simulink model "gm_uz_sixphase_VSD_transformation"  (R2021b)
settings: Solver=FixedStepAuto  StartTime=0.0  StopTime=inf  RelTol=1e-3
undefined symbols (not defined in the file or in its folder): a, b, c
libraries: hdlsllib x42, simulink x26, hdlmdlgenlib x20, dspsigops x6
(part 2 of 4)

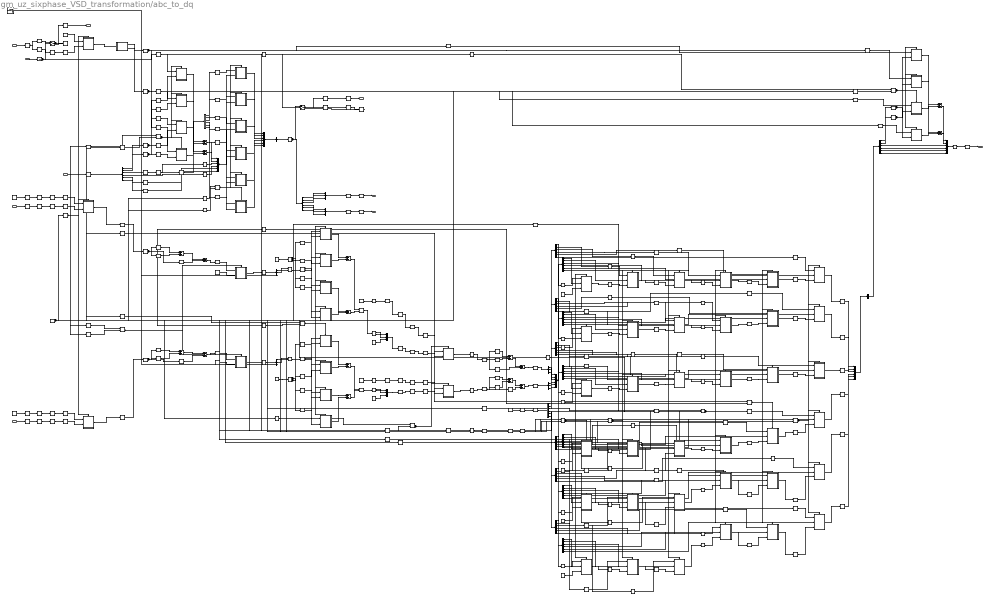
== system gm_uz_sixphase_VSD_transformation/abc_to_dq ==
  note: sin/cos calculation
  note: VSD and Park transformation
  note: VSD and Park inverse transformation
  note: Trigger Output
  x_in_dq : Inport  OutDataTypeStr=fixdt(1, 27, 18)  PortDimensions=[6]  SampleTime=1e-08
  theta_el : Inport  Port=2  OutDataTypeStr=fixdt(1, 18, 14)  PortDimensions=1  SampleTime=1e-08
  trigger_new_values : Inport  Port=3  OutDataTypeStr=boolean  PortDimensions=1  SampleTime=1e-08
  x_abc1_ll_pl : Inport  Port=4  OutDataTypeStr=fixdt(1, 27, 16)  PortDimensions=[3]  SampleTime=1e-08
  x_abc2_ll_pl : Inport  Port=5  OutDataTypeStr=fixdt(1, 27, 16)  PortDimensions=[3]  SampleTime=1e-08
  Add : Sum  AccumDataTypeStr=fixdt(1, 28, 16)  OutDataTypeStr=fixdt(1, 27, 16)  SampleTime=1e-10
  Add1 : Sum  AccumDataTypeStr=fixdt(1, 28, 18)  OutDataTypeStr=fixdt(1, 27, 18)  SampleTime=1e-10
  Add11 : Sum  Inputs=+-  AccumDataTypeStr=fixdt(1, 28, 16)  OutDataTypeStr=fixdt(1, 27, 16)  SampleTime=1e-10
  Add2 : Sum  Inputs=+-  AccumDataTypeStr=fixdt(1, 28, 18)  OutDataTypeStr=fixdt(1, 27, 18)  SampleTime=1e-10
  Complex to Real-Imag : ComplexToRealImag  SampleTime=1e-10
  Complex to Real-Imag1 : ComplexToRealImag  SampleTime=1e-10
  Constant : Constant  Value=0  OutDataTypeStr=fixdt(1, 27, 16)  SampleTime=1e-10
  Constant1 : Constant  Value=[1;-0.5;-0.5;0.86602783203125;-0.86602783203125;0;0;0.86602783203125;-0.86602783203125;0.5;0.5;-1;1;-0.5;-0.5;-0.86602783203125;0.86602783203125;0;0;-0.86602783203125;0.86602783203125;0.5;0.5;-1;1;1;1;0;0;0;0;0;0;1;1;1]  OutDataTypeStr=fixdt(1, 18, 16)  SampleTime=1e-10
  Constant11 : Constant  Value=[0.33333587646484375;0;0.33333587646484375;0;0.33333587646484375;0;-0.16666412353515625;0.28867340087890625;-0.16666412353515625;-0.28867340087890625;0.33333587646484375;0;-0.16666412353515625;-0.28867340087890625;-0.16666412353515625;0.28867340087890625;0.33333587646484375;0;0.28867340087890625;0.16666412353515625;-0.28867340087890625;0.16666412353515625;0;0.33333587646484375;-0.28867340087890625;0.16666412353515625;0.28867340087890625;0.16666412353515625;0;0.33333587646484375;0;-0.33333587646484375;0;-0.33333587646484375;0;0.33333587646484375]  OutDataTypeStr=fixdt(1, 18, 17)  SampleTime=1e-10
  Constant12 : Constant  Value="fi(0,1,18,16,\"hex\",\"08000 + 3b619 i\")"  OutDataTypeStr=fixdt(1, 18, 16)  SampleTime=1e-10
  Constant13 : Constant  Value="fi(0,1,18,16,\"hex\",\"08000 + 3b619 i\")"  OutDataTypeStr=fixdt(1, 18, 16)  SampleTime=1e-10
  Constant2 : Constant  Value=0  OutDataTypeStr=fixdt(1, 27, 16)  SampleTime=1e-10
  Delay9 : RateTransition  OutPortSampleTimeOpt=Multiple of input port sample time  OutPortSampleTimeMultiple=100
  Demux1_mux_1 : Mux  Inputs=3
  Demux1_mux_2 : Mux  Inputs=3
  Demux1_out1 : Delay  DelayLength=double(1)  InitialCondition=0  SampleTime=1e-10
  Demux1_out2 : Delay  DelayLength=double(1)  InitialCondition=0  SampleTime=1e-10
  Divide : Subsystem
      settings: MinAlgLoopOccurrences=on
  Divide1 : Subsystem
      settings: MinAlgLoopOccurrences=on
  Divide11 : Subsystem
      settings: MinAlgLoopOccurrences=on
  Divide2 : Subsystem
      settings: MinAlgLoopOccurrences=on
  Divide21 : Subsystem
      settings: MinAlgLoopOccurrences=on
  Divide3 : Subsystem
      settings: MinAlgLoopOccurrences=on
  Divide31 : Subsystem
      settings: MinAlgLoopOccurrences=on
  Divide4 : Subsystem
      settings: MinAlgLoopOccurrences=on
  From{,1..3,11..12,17..18,21..22} (10 alike) : hdlmdlgenlib/Buffer
      settings: SourceProductBaseCode=SL
  Gain : Subsystem
      settings: MinAlgLoopOccurrences=on
  Gain2 : Subsystem
      settings: MinAlgLoopOccurrences=on
  Gain21 : Subsystem
      settings: MinAlgLoopOccurrences=on
  Gain2_const : Constant  Value=0.6666717529296875  OutDataTypeStr=fixdt(1, 18, 16)  SampleTime=1e-10
  Gain2_const1 : Constant  Value=0.6666717529296875  OutDataTypeStr=fixdt(1, 18, 16)  SampleTime=1e-10
  Gain2_out_dtc : DataTypeConversion  OutDataTypeStr=fixdt(1, 27, 16)  SampleTime=1e-10  SaturateOnIntegerOverflow=on
  Gain2_out_dtc1 : DataTypeConversion  OutDataTypeStr=fixdt(1, 27, 16)  SampleTime=1e-10  SaturateOnIntegerOverflow=on
  Gain4_const : Constant  Value=[1;0;0.5;-0.5;0.86602783203125;0.5;-0.5;-0.86602783203125;0.5]  OutDataTypeStr=fixdt(1, 18, 16)  SampleTime=1e-10
  Gain4_const1 : Constant  Value=[1;-0.5;-0.5;0;0.86602783203125;-0.86602783203125;1;1;1]  OutDataTypeStr=fixdt(1, 18, 16)  SampleTime=1e-10
  Gain4_const2 : Constant  Value=[1;0;0.5;-0.5;0.86602783203125;0.5;-0.5;-0.86602783203125;0.5]  OutDataTypeStr=fixdt(1, 18, 16)  SampleTime=1e-10
  Gain4_const3 : Constant  Value=[1;-0.5;-0.5;0;0.86602783203125;-0.86602783203125;1;1;1]  OutDataTypeStr=fixdt(1, 18, 16)  SampleTime=1e-10
  Gain_const : Constant  Value=0.1591548919677734375  OutDataTypeStr=fixdt(1, 18, 19)  SampleTime=1e-10
  Goto : hdlmdlgenlib/Buffer
      settings: SourceProductBaseCode=SL
  Goto1 : hdlmdlgenlib/Buffer
      settings: SourceProductBaseCode=SL
  Goto2 : hdlmdlgenlib/Buffer
      settings: SourceProductBaseCode=SL
  MMul_add_01 : Sum  OutDataTypeStr=fixdt(1, 27, 16)  SaturateOnIntegerOverflow=on  SampleTime=1e-10
  MMul_add_011 : Sum  OutDataTypeStr=fixdt(1, 27, 16)  SaturateOnIntegerOverflow=on  SampleTime=1e-10
  MMul_add_012 : Sum  OutDataTypeStr=fixdt(1, 27, 16)  SaturateOnIntegerOverflow=on  SampleTime=1e-10
  MMul_add_013 : Sum  OutDataTypeStr=fixdt(1, 27, 16)  SaturateOnIntegerOverflow=on  SampleTime=1e-10
  MMul_add_{12,121..123} (4 alike) : Sum  OutDataTypeStr=fixdt(1, 27, 16)  SaturateOnIntegerOverflow=on  SampleTime=1e-10
  MMul_dot_product : Subsystem
      settings: MinAlgLoopOccurrences=on
  MMul_dot_product1 : Subsystem
      settings: MinAlgLoopOccurrences=on
  MMul_dot_product2 : Subsystem
      settings: MinAlgLoopOccurrences=on
  MMul_dot_product3 : Subsystem
      settings: MinAlgLoopOccurrences=on
  MMul_dot_product_out_dtc{,1..3} (4 alike) : DataTypeConversion  OutDataTypeStr=fixdt(1, 27, 16)  SampleTime=1e-10  SaturateOnIntegerOverflow=on
  MatrixMultiply_out1_0_wire : hdlmdlgenlib/Buffer
      settings: SourceProductBaseCode=SL
  MatrixMultiply_out1_1_wire : hdlmdlgenlib/Buffer
      settings: SourceProductBaseCode=SL
  Product : Subsystem
      settings: MinAlgLoopOccurrences=on
  Product1 : Subsystem
      settings: MinAlgLoopOccurrences=on
  Product2 : Subsystem
      settings: MinAlgLoopOccurrences=on
  Product3 : Subsystem
      settings: MinAlgLoopOccurrences=on
  Product4 : Subsystem
      settings: MinAlgLoopOccurrences=on
  Product5 : Subsystem
      settings: MinAlgLoopOccurrences=on
  Product6 : Subsystem
      settings: MinAlgLoopOccurrences=on
  Product7 : Subsystem
      settings: MinAlgLoopOccurrences=on
  Product_AC_minus_BD : Sum  Inputs=+-  OutDataTypeStr=fixdt(1, 27, 16)  SampleTime=1e-10
  Product_AC_minus_BD1 : Sum  Inputs=+-  OutDataTypeStr=fixdt(1, 27, 16)  SampleTime=1e-10
  Product_AD_plus_BC : Sum  OutDataTypeStr=fixdt(1, 27, 16)  SampleTime=1e-10
  Product_AD_plus_BC1 : Sum  OutDataTypeStr=fixdt(1, 27, 16)  SampleTime=1e-10
  Product_C2ReIm_{1..2,11,21} (4 alike) : ComplexToRealImag  SampleTime=1e-10
  Product_ReIm2Complex : RealImagToComplex  SampleTime=1e-10
  Product_ReIm2Complex1 : RealImagToComplex  SampleTime=1e-10
  Real-Imag to Complex : RealImagToComplex  ConstantPart="fi(0,1,27,16,\"hex\",\"0000000\")"  SampleTime=1e-10
  Real-Imag to Complex1 : RealImagToComplex  ConstantPart="fi(0,1,27,16,\"hex\",\"0000000\")"  SampleTime=1e-10
  Reshape{,1..3} (4 alike) : Reshape  OutputDimensionality=Column vector (2-D)
  Row2Col_in{0..1,11..13} (5 alike) : Reshape  OutputDimensionality=Column vector (2-D)
  Row2Col_in01 : Reshape  OutputDimensionality=Column vector (2-D)
  Row2Col_in02 : Reshape  OutputDimensionality=Column vector (2-D)
  Row2Col_in03 : Reshape  OutputDimensionality=Column vector (2-D)
  Sine HDL Optimized : Subsystem  mask(Sine and Cosine HDL optimized block){OutputFormula=sin(2*pi*u) and cos(2*pi*u), NumDataPoints=double(256), TableDataTypeStr=fixdt(0,17,16), SimulateLUTROMDelay=off}
      mask prompts: OutputFormula "Simulink:masks:OutputFormula_MP"; NumDataPoints "HDLShared:hdlshared:CosineHDL_Npts"; TableDataTypeStr "Simulink:blkprm_prompts:TABLE_UNIFIEDDATATYPE"; SimulateLUTROMDelay "HDLShared:hdlshared:CosineHDL_SimulateLUTDelay"
      mask help: Sine and Cosine HDL optimized block using quarter wave symmetry, and HDL friendly settings.
      mask Help: helpview([docroot '/hdlcoder/helptargets.map'],'SineAndCosineHDL_Optimized');
      mask TypeOptions OutputFormula: sin(2*pi*u) | cos(2*pi*u) | exp(j*2*pi*u) | sin(2*pi*u) and cos(2*pi*u)
      mask Display:
      | port_label('input',1,'u')
      | port_label('output',1,'sin(2*pi*u)')
      | port_label('output',2,'cos(2*pi*u)')
      | xpos = 0.35;
      | yoffset = 0.5;
      | if ( SimulateLUTROMDelay )
      |   text(xpos,yoffset,'HDL (Z^{-1})','texmode','on')
      | else
      |    text(xpos,yoffset,'HDL')
      | end
  Switch : Switch  Criteria=u2 ~= 0  Threshold=double(0)  OutDataTypeStr=fixdt(1, 27, 18)  SampleTime=1e-10
  Switch1 : Switch  Criteria=u2 ~= 0  Threshold=double(0)  OutDataTypeStr=fixdt(1, 18, 14)  SampleTime=1e-08
  Switch_out1 : Delay  DelayLength=double(1)  InitialCondition=0  SampleTime=1e-10
  Switch_out11 : Delay  DelayLength=double(1)  InitialCondition=0  SampleTime=1e-10
  Transformation_out1 : Delay  DelayLength=double(1)  InitialCondition=0  SampleTime=1e-10
  Unit Delay : UnitDelay  SampleTime=1e-08
  _adder_MultiplyAdd : Subsystem
      settings: MinAlgLoopOccurrences=on
  _adder_MultiplyAdd1 : Subsystem
      settings: MinAlgLoopOccurrences=on
  _adder_MultiplyAdd10 : Subsystem
      settings: MinAlgLoopOccurrences=on
  _adder_MultiplyAdd11 : Subsystem
      settings: MinAlgLoopOccurrences=on
  _adder_MultiplyAdd12 : Subsystem
      settings: MinAlgLoopOccurrences=on
  _adder_MultiplyAdd13 : Subsystem
      settings: MinAlgLoopOccurrences=on
  _adder_MultiplyAdd14 : Subsystem
      settings: MinAlgLoopOccurrences=on
  _adder_MultiplyAdd15 : Subsystem
      settings: MinAlgLoopOccurrences=on
  _adder_MultiplyAdd16 : Subsystem
      settings: MinAlgLoopOccurrences=on
  _adder_MultiplyAdd17 : Subsystem
      settings: MinAlgLoopOccurrences=on
  _adder_MultiplyAdd18 : Subsystem
      settings: MinAlgLoopOccurrences=on
  _adder_MultiplyAdd19 : Subsystem
      settings: MinAlgLoopOccurrences=on
  _adder_MultiplyAdd2 : Subsystem
      settings: MinAlgLoopOccurrences=on
  _adder_MultiplyAdd20 : Subsystem
      settings: MinAlgLoopOccurrences=on
  _adder_MultiplyAdd21 : Subsystem
      settings: MinAlgLoopOccurrences=on
  _adder_MultiplyAdd22 : Subsystem
      settings: MinAlgLoopOccurrences=on
  _adder_MultiplyAdd23 : Subsystem
      settings: MinAlgLoopOccurrences=on
  _adder_MultiplyAdd24 : Subsystem
      settings: MinAlgLoopOccurrences=on
  _adder_MultiplyAdd25 : Subsystem
      settings: MinAlgLoopOccurrences=on
  _adder_MultiplyAdd26 : Subsystem
      settings: MinAlgLoopOccurrences=on
  _adder_MultiplyAdd27 : Subsystem
      settings: MinAlgLoopOccurrences=on
  _adder_MultiplyAdd28 : Subsystem
      settings: MinAlgLoopOccurrences=on
  _adder_MultiplyAdd29 : Subsystem
      settings: MinAlgLoopOccurrences=on
  _adder_MultiplyAdd3 : Subsystem
      settings: MinAlgLoopOccurrences=on
  _adder_MultiplyAdd30 : Subsystem
      settings: MinAlgLoopOccurrences=on
  _adder_MultiplyAdd31 : Subsystem
      settings: MinAlgLoopOccurrences=on
  _adder_MultiplyAdd32 : Subsystem
      settings: MinAlgLoopOccurrences=on
  _adder_MultiplyAdd33 : Subsystem
      settings: MinAlgLoopOccurrences=on
  _adder_MultiplyAdd34 : Subsystem
      settings: MinAlgLoopOccurrences=on
  _adder_MultiplyAdd35 : Subsystem
      settings: MinAlgLoopOccurrences=on
  _adder_MultiplyAdd4 : Subsystem
      settings: MinAlgLoopOccurrences=on
  _adder_MultiplyAdd5 : Subsystem
      settings: MinAlgLoopOccurrences=on
  _adder_MultiplyAdd6 : Subsystem
      settings: MinAlgLoopOccurrences=on
  _adder_MultiplyAdd7 : Subsystem
      settings: MinAlgLoopOccurrences=on
  _adder_MultiplyAdd8 : Subsystem
      settings: MinAlgLoopOccurrences=on
  _adder_MultiplyAdd9 : Subsystem
      settings: MinAlgLoopOccurrences=on
  _adder_MultiplyAdd_out_dtc{,1..35} (36 alike) : DataTypeConversion  OutDataTypeStr=fixdt(1, 27, 16)  SampleTime=1e-10
  _bias{,1..5} (6 alike) : Constant  Value=double(0)  OutDataTypeStr=fixdt(1, 27, 16)  SampleTime=1e-10
  abc   to   alpha_beta_0_out1_2_term2 : Terminator
  abc   to   alpha_beta_0_out1_2_term21 : Terminator
  crp_temp_MAC : Subsystem
      settings: MinAlgLoopOccurrences=on
  crp_temp_MAC1 : Subsystem
      settings: MinAlgLoopOccurrences=on
  crp_temp_MAC2 : Subsystem
      settings: MinAlgLoopOccurrences=on
  crp_temp_MAC3 : Subsystem
      settings: MinAlgLoopOccurrences=on
  crp_temp_MAC4 : Subsystem
      settings: MinAlgLoopOccurrences=on
  crp_temp_MAC5 : Subsystem
      settings: MinAlgLoopOccurrences=on
  ctr_99 : simulink/Sources/Counter Limited  uplimit=double(99)  tsamp=1e-10
  delayMatch : Delay  DelayLength=double(1)  InitialCondition=0  SampleTime=1e-08
  delayMatch1 : Delay  DelayLength=double(1)  InitialCondition=0  SampleTime=1e-08
  delayMatch{2..61} (60 alike) : Delay  DelayLength=double(1)  InitialCondition=0  SampleTime=1e-10
  delayMatch62 : Delay  DelayLength=double(1)  InitialCondition=0  SampleTime=1e-08
  enb_counter_ge_11 : simulink/Logic and Bit Operations/Compare To Constant  relop=>=  const=double(11)  OutDataTypeStr=boolean
  enb_counter_ge_11_and_enb_counter_le_14 : Logic  AllPortsSameDT=off  OutDataTypeStr=boolean  SampleTime=1e-10
  enb_counter_ge_14 : simulink/Logic and Bit Operations/Compare To Constant  relop=>=  const=double(14)  OutDataTypeStr=boolean
  enb_counter_ge_14_and_enb_counter_le_17 : Logic  AllPortsSameDT=off  OutDataTypeStr=boolean  SampleTime=1e-10
  enb_counter_ge_17 : simulink/Logic and Bit Operations/Compare To Constant  relop=>=  const=double(17)  OutDataTypeStr=boolean
  enb_counter_ge_17_and_enb_counter_le_20 : Logic  AllPortsSameDT=off  OutDataTypeStr=boolean  SampleTime=1e-10
  enb_counter_ge_2 : simulink/Logic and Bit Operations/Compare To Constant  relop=>=  const=double(2)  OutDataTypeStr=boolean
  enb_counter_ge_20 : simulink/Logic and Bit Operations/Compare To Constant  relop=>=  const=double(20)  OutDataTypeStr=boolean
  enb_counter_ge_20_and_enb_counter_le_23 : Logic  AllPortsSameDT=off  OutDataTypeStr=boolean  SampleTime=1e-10
  enb_counter_ge_23 : simulink/Logic and Bit Operations/Compare To Constant  relop=>=  const=double(23)  OutDataTypeStr=boolean
  enb_counter_ge_23_and_enb_counter_le_26 : Logic  AllPortsSameDT=off  OutDataTypeStr=boolean  SampleTime=1e-10
  enb_counter_ge_26 : simulink/Logic and Bit Operations/Compare To Constant  relop=>=  const=double(26)  OutDataTypeStr=boolean
  enb_counter_ge_26_and_enb_counter_le_28 : Logic  AllPortsSameDT=off  OutDataTypeStr=boolean  SampleTime=1e-10
  enb_counter_ge_2_and_enb_counter_le_4 : Logic  AllPortsSameDT=off  OutDataTypeStr=boolean  SampleTime=1e-10
  enb_counter_ge_3 : simulink/Logic and Bit Operations/Compare To Constant  relop=>=  const=double(3)  OutDataTypeStr=boolean
  enb_counter_ge_3_and_enb_counter_le_5 : Logic  AllPortsSameDT=off  OutDataTypeStr=boolean  SampleTime=1e-10
  enb_counter_ge_4 : simulink/Logic and Bit Operations/Compare To Constant  relop=>=  const=double(4)  OutDataTypeStr=boolean
  enb_counter_ge_4_and_enb_counter_le_6 : Logic  AllPortsSameDT=off  OutDataTypeStr=boolean  SampleTime=1e-10
  enb_counter_ge_5 : simulink/Logic and Bit Operations/Compare To Constant  relop=>=  const=double(5)  OutDataTypeStr=boolean
  enb_counter_ge_5_and_enb_counter_le_10 : Logic  AllPortsSameDT=off  OutDataTypeStr=boolean  SampleTime=1e-10
  enb_counter_ge_6 : simulink/Logic and Bit Operations/Compare To Constant  relop=>=  const=double(6)  OutDataTypeStr=boolean
  enb_counter_ge_6_and_enb_counter_le_8 : Logic  AllPortsSameDT=off  OutDataTypeStr=boolean  SampleTime=1e-10
  enb_counter_ge_8 : simulink/Logic and Bit Operations/Compare To Constant  relop=>=  const=double(8)  OutDataTypeStr=boolean
  enb_counter_ge_8_and_enb_counter_le_11 : Logic  AllPortsSameDT=off  OutDataTypeStr=boolean  SampleTime=1e-10
  enb_counter_le_10 : simulink/Logic and Bit Operations/Compare To Constant  relop=<=  const=double(10)  OutDataTypeStr=boolean
  enb_counter_le_11 : simulink/Logic and Bit Operations/Compare To Constant  relop=<=  const=double(11)  OutDataTypeStr=boolean
  enb_counter_le_14 : simulink/Logic and Bit Operations/Compare To Constant  relop=<=  const=double(14)  OutDataTypeStr=boolean
  enb_counter_le_17 : simulink/Logic and Bit Operations/Compare To Constant  relop=<=  const=double(17)  OutDataTypeStr=boolean
  enb_counter_le_2 : simulink/Logic and Bit Operations/Compare To Constant  relop=<=  const=double(2)  OutDataTypeStr=boolean
  enb_counter_le_20 : simulink/Logic and Bit Operations/Compare To Constant  relop=<=  const=double(20)  OutDataTypeStr=boolean
  enb_counter_le_23 : simulink/Logic and Bit Operations/Compare To Constant  relop=<=  const=double(23)  OutDataTypeStr=boolean
  enb_counter_le_26 : simulink/Logic and Bit Operations/Compare To Constant  relop=<=  const=double(26)  OutDataTypeStr=boolean
  enb_counter_le_28 : simulink/Logic and Bit Operations/Compare To Constant  relop=<=  const=double(28)  OutDataTypeStr=boolean
  enb_counter_le_4 : simulink/Logic and Bit Operations/Compare To Constant  relop=<=  const=double(4)  OutDataTypeStr=boolean
  enb_counter_le_5 : simulink/Logic and Bit Operations/Compare To Constant  relop=<=  const=double(5)  OutDataTypeStr=boolean
  enb_counter_le_6 : simulink/Logic and Bit Operations/Compare To Constant  relop=<=  const=double(6)  OutDataTypeStr=boolean
  enb_counter_le_8 : simulink/Logic and Bit Operations/Compare To Constant  relop=<=  const=double(8)  OutDataTypeStr=boolean
  in0_repeat : dspsigops/Repeat  N=double(100)  RateOptions=Allow multirate processing  ic=0  mode=Unused parameter value
  in1_repeat : dspsigops/Repeat  N=double(100)  RateOptions=Allow multirate processing  ic=0  mode=Unused parameter value
  in2_repeat : dspsigops/Repeat  N=double(100)  RateOptions=Allow multirate processing  ic=0  mode=Unused parameter value
  in3_repeat : dspsigops/Repeat  N=double(100)  RateOptions=Allow multirate processing  ic=0  mode=Unused parameter value
  in4_repeat : dspsigops/Repeat  N=double(100)  RateOptions=Allow multirate processing  ic=0  mode=Unused parameter value
  in5_repeat : dspsigops/Repeat  N=double(100)  RateOptions=Allow multirate processing  ic=0  mode=Unused parameter value
  inverse Transformation_out1 : hdlmdlgenlib/Buffer
      settings: SourceProductBaseCode=SL
  mux : Mux  Inputs=3
  mux1 : Mux  Inputs=3
  mux2 : Mux  Inputs=6
  mux3 : Mux  Inputs=6
  mux4 : Mux  Inputs=6
  reshape_dotProduct{,1..3} (4 alike) : Reshape  OutputDimensionality=Customize  OutputDimensions=[3,3]
  reshape_mmulResult{,1..3} (4 alike) : Reshape  OutputDimensionality=Customize  OutputDimensions=[3,1]
  select_0 : Selector  NumberOfDimensions=2  SampleTime=1e-10  IndexOptions=Index vector (dialog),Select all  Indices=double(1),[]  OutputSizes=1
  select_01 : Selector  NumberOfDimensions=2  SampleTime=1e-10  IndexOptions=Index vector (dialog),Select all  Indices=double(1),[]  OutputSizes=1
  select_02 : Selector  NumberOfDimensions=2  SampleTime=1e-10  IndexOptions=Index vector (dialog),Select all  Indices=double(1),[]  OutputSizes=1
  select_03 : Selector  NumberOfDimensions=2  SampleTime=1e-10  IndexOptions=Index vector (dialog),Select all  Indices=double(1),[]  OutputSizes=1
  select_{1,11..13} (4 alike) : Selector  NumberOfDimensions=2  SampleTime=1e-10  IndexOptions=Index vector (dialog),Select all  Indices=double(2),[]  OutputSizes=1
  select_{2,21..23} (4 alike) : Selector  NumberOfDimensions=2  SampleTime=1e-10  IndexOptions=Index vector (dialog),Select all  Indices=double(3),[]  OutputSizes=1
  select_indices0 : Selector  SampleTime=1e-10  IndexOptions=Index vector (dialog)  Indices=double([1 4 7 2 5 8 3 6 9])  OutputSizes=1
  select_indices01 : Selector  SampleTime=1e-10  IndexOptions=Index vector (dialog)  Indices=double([1 4 7 2 5 8 3 6 9])  OutputSizes=1
  select_indices02 : Selector  SampleTime=1e-10  IndexOptions=Index vector (dialog)  Indices=double([1 4 7 2 5 8 3 6 9])  OutputSizes=1
  select_indices03 : Selector  SampleTime=1e-10  IndexOptions=Index vector (dialog)  Indices=double([1 4 7 2 5 8 3 6 9])  OutputSizes=1
  select_indices{1,11..13} (4 alike) : Selector  SampleTime=1e-10  IndexOptions=Index vector (dialog)  Indices=double([1 2 3 1 2 3 1 2 3])  OutputSizes=1
  t{,5..6,21..32} (15 alike) : Demux  Outputs=6
  t{1..4} (4 alike) : Demux  Outputs=3
  t{9..12} (4 alike) : Reshape  OutputDimensionality=Customize  OutputDimensions=[3,3]
  t13 : Math  Operator=transpose  SaturateOnIntegerOverflow=on
  t14 : Subsystem
  t15 : Mux  Inputs=6
  t16 : Concatenate  NumInputs=1  Mode=Multidimensional array  ConcatenateDimension=2
  t17 : Math  Operator=transpose  SaturateOnIntegerOverflow=on
  t18 : Subsystem
  t19 : Mux  Inputs=6
  t20 : Concatenate  NumInputs=1  Mode=Multidimensional array  ConcatenateDimension=2
  t{33..36} (4 alike) : RateTransition  OutPortSampleTimeOpt=Multiple of input port sample time  OutPortSampleTimeMultiple=100
  t7 : Reshape  OutputDimensionality=Customize  OutputDimensions=[6,6]
  t8 : Reshape  OutputDimensionality=Customize  OutputDimensions=[6,6]
  vectorized_in0 : Reshape  OutputDimensionality=Row vector (2-D)
  vectorized_in01 : Reshape  OutputDimensionality=Row vector (2-D)
  vectorized_in02 : Reshape  OutputDimensionality=Row vector (2-D)
  vectorized_in03 : Reshape  OutputDimensionality=Row vector (2-D)
  x_in_dq_0_wire : hdlmdlgenlib/Buffer
      settings: SourceProductBaseCode=SL
  x_in_dq_1_wire : hdlmdlgenlib/Buffer
      settings: SourceProductBaseCode=SL
  theta_el_axi : Outport  SampleTime=1e-08
  x_abc_out_axi : Outport  Port=2  SampleTime=1e-08
  x_abc_1 : Outport  Port=3  SampleTime=1e-08
  x_abc_2 : Outport  Port=4  SampleTime=1e-08
  x_out_dq : Outport  Port=5  SampleTime=1e-08
  wires:
  x_in_dq/1 -> in2_repeat/1
  theta_el/1 -> Goto2/1
  trigger_new_values/1 -> Unit Delay/1
  x_abc1_ll_pl/1 -> in4_repeat/1
  x_abc2_ll_pl/1 -> in5_repeat/1
  delayMatch1/1 -> in3_repeat/1
  Unit Delay/1 -> Switch1/2, in0_repeat/1
  delayMatch62/1 -> theta_el_axi/1
  t33/1 -> x_abc_1/1
  t34/1 -> x_abc_2/1
  t35/1 -> x_abc_out_axi/1
  t36/1 -> x_out_dq/1
  Switch1/1 -> delayMatch62/1, delayMatch/1
  delayMatch/1 -> Switch1/3
  Delay9/1 -> in1_repeat/1
  Goto2/1 -> From1/1, From/1
  From1/1 -> Switch1/1
  From/1 -> delayMatch1/1
  Demux1_out1/1 -> t33/1
  Demux1_out2/1 -> t34/1
  Switch_out1/1 -> Delay9/1
  Switch_out11/1 -> t35/1
  Transformation_out1/1 -> t36/1
  in0_repeat/1 -> Switch/2
  in1_repeat/1 -> Switch/3
  in2_repeat/1 -> t/1
  in3_repeat/1 -> Gain/2(in1)
  in4_repeat/1 -> Reshape/1
  in5_repeat/1 -> Reshape2/1
  t7/1 -> t17/1
  Divide1/1(out0) -> Add/2
  From21/1 -> Divide3/1(in0)
  Divide3/1(out0) -> Add1/2
  Add1/1 -> mux4/2
  From11/1 -> Divide2/1(in0)
  Divide2/1(out0) -> Add1/1
  delayMatch2/1 -> Divide4/2(in1)
  delayMatch4/1 -> Divide11/2(in1)
  delayMatch6/1 -> mux4/3
  delayMatch7/1 -> mux4/4
  delayMatch8/1 -> mux4/5
  delayMatch9/1 -> mux4/6
  Divide11/1(out0) -> Add2/2
  From18/1 -> Divide11/1(in0)
  Gain/1(out0) -> Sine HDL Optimized/1(u)
  Sine HDL Optimized/1(x) -> Goto/1
  Sine HDL Optimized/2(y) -> Goto1/1
  Goto/1 -> From3/1, From12/1, From18/1, From11/1
  Divide21/1(out0) -> Add11/2
  t8/1 -> t13/1
  Reshape/1 -> select_indices1/1
  reshape_mmulResult/1 -> Gain2/1(in0)
  Gain2_out_dtc/1 -> t1/1
  Real-Imag to Complex/1 -> Product_C2ReIm_1/1
  Constant12/1 -> Product_C2ReIm_2/1
  Product_ReIm2Complex/1 -> Complex to Real-Imag/1
  Complex to Real-Imag/1 -> mux/1
  Complex to Real-Imag/2 -> mux/2
  Constant/1 -> mux/3
  mux/1 -> Reshape1/1
  Reshape1/1 -> select_indices11/1
  reshape_mmulResult1/1 -> t3/1
  Reshape2/1 -> select_indices12/1
  reshape_mmulResult2/1 -> Gain21/1(in0)
  Gain2_out_dtc1/1 -> t2/1
  Real-Imag to Complex1/1 -> Product_C2ReIm_11/1
  Constant13/1 -> Product_C2ReIm_21/1
  Product_ReIm2Complex1/1 -> Complex to Real-Imag1/1
  Complex to Real-Imag1/1 -> mux1/1
  Complex to Real-Imag1/2 -> mux1/2
  Constant2/1 -> mux1/3
  mux1/1 -> Reshape3/1
  Reshape3/1 -> select_indices13/1
  reshape_mmulResult3/1 -> t4/1
  mux2/1 -> t32/1, t30/1, t28/1, t26/1, t24/1, t22/1
  t16/1 -> t5/1
  MatrixMultiply_out1_0_wire/1 -> Divide/2(in1), Divide21/2(in1)
  MatrixMultiply_out1_1_wire/1 -> Divide1/2(in1), Divide31/2(in1)
  Divide/1(out0) -> Add/1
  Add/1 -> mux3/1
  mux3/1 -> Transformation_out1/1
  Add11/1 -> mux3/2
  Divide31/1(out0) -> Add11/1
  Goto1/1 -> From22/1, From2/1, From21/1, From17/1
  From17/1 -> Divide4/1(in0)
  Divide4/1(out0) -> Add2/1
  Add2/1 -> mux4/1
  mux4/1 -> crp_temp_MAC1/2(in1), crp_temp_MAC2/2(in1), crp_temp_MAC/2(in1), crp_temp_MAC3/2(in1), crp_temp_MAC5/2(in1), crp_temp_MAC4/2(in1)
  t20/1 -> inverse Transformation_out1/1
  inverse Transformation_out1/1 -> t6/1, Switch/1
  t/1 -> x_in_dq_0_wire/1
  t/2 -> x_in_dq_1_wire/1
  t/3 -> delayMatch6/1
  t/4 -> delayMatch7/1
  t/5 -> delayMatch8/1
  t/6 -> delayMatch9/1
  t1/1 -> Real-Imag to Complex/1
  t1/2 -> Real-Imag to Complex/2
  t1/3 -> abc   to   alpha_beta_0_out1_2_term2/1
  t2/1 -> Real-Imag to Complex1/1
  t2/2 -> Real-Imag to Complex1/2
  t2/3 -> abc   to   alpha_beta_0_out1_2_term21/1
  t3/1 -> mux2/1
  t3/2 -> mux2/2
  t3/3 -> mux2/3
  t4/1 -> mux2/4
  t4/2 -> mux2/5
  t4/3 -> mux2/6
  t5/1 -> MatrixMultiply_out1_0_wire/1
  t5/2 -> MatrixMultiply_out1_1_wire/1
  t5/3 -> mux3/3
  t5/4 -> mux3/4
  t5/5 -> mux3/5
  t5/6 -> mux3/6
  t6/1 -> Demux1_mux_1/1
  t6/2 -> Demux1_mux_1/2
  t6/3 -> Demux1_mux_1/3
  t6/4 -> Demux1_mux_2/1
  t6/5 -> Demux1_mux_2/2
  t6/6 -> Demux1_mux_2/3
  Constant1/1 -> t7/1
  Constant11/1 -> t8/1
  t9/1 -> vectorized_in0/1
  vectorized_in0/1 -> select_indices0/1
  select_indices0/1 -> Row2Col_in0/1
  select_indices1/1 -> Row2Col_in1/1
  Row2Col_in0/1 -> MMul_dot_product/1(in0)
  Row2Col_in1/1 -> MMul_dot_product/2(in1)
  MMul_dot_product_out_dtc/1 -> reshape_dotProduct/1
  reshape_dotProduct/1 -> select_2/1, select_1/1, select_0/1
  select_0/1 -> MMul_add_01/1
  select_1/1 -> MMul_add_01/2
  MMul_add_01/1 -> MMul_add_12/1
  select_2/1 -> MMul_add_12/2
  MMul_add_12/1 -> reshape_mmulResult/1
  Gain4_const/1 -> t9/1
  t10/1 -> vectorized_in01/1
  vectorized_in01/1 -> select_indices01/1
  select_indices01/1 -> Row2Col_in01/1
  select_indices11/1 -> Row2Col_in11/1
  delayMatch20/1 -> MMul_dot_product1/1(in0)
  Row2Col_in11/1 -> MMul_dot_product1/2(in1)
  MMul_dot_product_out_dtc1/1 -> reshape_dotProduct1/1
  reshape_dotProduct1/1 -> select_21/1, select_11/1, select_01/1
  select_01/1 -> MMul_add_011/1
  select_11/1 -> MMul_add_011/2
  MMul_add_011/1 -> MMul_add_121/1
  select_21/1 -> MMul_add_121/2
  MMul_add_121/1 -> reshape_mmulResult1/1
  Gain4_const1/1 -> t10/1
  t11/1 -> vectorized_in02/1
  vectorized_in02/1 -> select_indices02/1
  select_indices02/1 -> Row2Col_in02/1
  select_indices12/1 -> Row2Col_in12/1
  Row2Col_in02/1 -> MMul_dot_product2/1(in0)
  Row2Col_in12/1 -> MMul_dot_product2/2(in1)
  MMul_dot_product_out_dtc2/1 -> reshape_dotProduct2/1
  reshape_dotProduct2/1 -> select_22/1, select_12/1, select_02/1
  select_02/1 -> MMul_add_012/1
  select_12/1 -> MMul_add_012/2
  MMul_add_012/1 -> MMul_add_122/1
  select_22/1 -> MMul_add_122/2
  MMul_add_122/1 -> reshape_mmulResult2/1
  Gain4_const2/1 -> t11/1
  t12/1 -> vectorized_in03/1
  vectorized_in03/1 -> select_indices03/1
  select_indices03/1 -> Row2Col_in03/1
  select_indices13/1 -> Row2Col_in13/1
  delayMatch25/1 -> MMul_dot_product3/1(in0)
  Row2Col_in13/1 -> MMul_dot_product3/2(in1)
  MMul_dot_product_out_dtc3/1 -> reshape_dotProduct3/1
  reshape_dotProduct3/1 -> select_23/1, select_13/1, select_03/1
  select_03/1 -> MMul_add_013/1
  select_13/1 -> MMul_add_013/2
  MMul_add_013/1 -> MMul_add_123/1
  select_23/1 -> MMul_add_123/2
  MMul_add_123/1 -> reshape_mmulResult3/1
  Gain4_const3/1 -> t12/1
  t13/1 -> t14/1(in0)
  t14/1(out0) -> t21/1
  t14/2(out1) -> t23/1
  t14/3(out2) -> t25/1
  t14/4(out3) -> t27/1
  t14/5(out4) -> t29/1
  t14/6(out5) -> t31/1
  _adder_MultiplyAdd_out_dtc5/1 -> t15/1
  _adder_MultiplyAdd_out_dtc11/1 -> t15/2
  _adder_MultiplyAdd_out_dtc17/1 -> t15/3
  _adder_MultiplyAdd_out_dtc23/1 -> t15/4
  _adder_MultiplyAdd_out_dtc29/1 -> t15/5
  _adder_MultiplyAdd_out_dtc35/1 -> t15/6
  t15/1 -> t16/1
  t17/1 -> t18/1(in0)
  delayMatch10/1 -> crp_temp_MAC1/1(in0)
  delayMatch11/1 -> crp_temp_MAC2/1(in0)
  delayMatch12/1 -> crp_temp_MAC/1(in0)
  delayMatch13/1 -> crp_temp_MAC3/1(in0)
  delayMatch14/1 -> crp_temp_MAC5/1(in0)
  delayMatch15/1 -> crp_temp_MAC4/1(in0)
  crp_temp_MAC1/1(out0) -> t19/1
  crp_temp_MAC2/1(out0) -> t19/2
  crp_temp_MAC/1(out0) -> t19/3
  crp_temp_MAC3/1(out0) -> t19/4
  crp_temp_MAC5/1(out0) -> t19/5
  crp_temp_MAC4/1(out0) -> t19/6
  t19/1 -> t20/1
  _bias/1 -> _adder_MultiplyAdd/3(in2)
  delayMatch26/1 -> _adder_MultiplyAdd/1(in0)
  t22/1 -> _adder_MultiplyAdd/2(in1)
  delayMatch27/1 -> _adder_MultiplyAdd1/1(in0)
  _adder_MultiplyAdd_out_dtc/1 -> _adder_MultiplyAdd1/3(in2)
  delayMatch28/1 -> _adder_MultiplyAdd2/1(in0)
  _adder_MultiplyAdd_out_dtc1/1 -> _adder_MultiplyAdd2/3(in2)
  delayMatch29/1 -> _adder_MultiplyAdd3/1(in0)
  _adder_MultiplyAdd_out_dtc2/1 -> _adder_MultiplyAdd3/3(in2)
  delayMatch30/1 -> _adder_MultiplyAdd4/1(in0)
  _adder_MultiplyAdd_out_dtc3/1 -> _adder_MultiplyAdd4/3(in2)
  delayMatch56/1 -> _adder_MultiplyAdd5/1(in0)
  _adder_MultiplyAdd_out_dtc4/1 -> _adder_MultiplyAdd5/3(in2)
  _bias1/1 -> _adder_MultiplyAdd6/3(in2)
  delayMatch31/1 -> _adder_MultiplyAdd6/1(in0)
  t24/1 -> _adder_MultiplyAdd6/2(in1)
  delayMatch32/1 -> _adder_MultiplyAdd7/1(in0)
  _adder_MultiplyAdd_out_dtc6/1 -> _adder_MultiplyAdd7/3(in2)
  delayMatch33/1 -> _adder_MultiplyAdd8/1(in0)
  _adder_MultiplyAdd_out_dtc7/1 -> _adder_MultiplyAdd8/3(in2)
  delayMatch34/1 -> _adder_MultiplyAdd9/1(in0)
  _adder_MultiplyAdd_out_dtc8/1 -> _adder_MultiplyAdd9/3(in2)
  delayMatch35/1 -> _adder_MultiplyAdd10/1(in0)
  _adder_MultiplyAdd_out_dtc9/1 -> _adder_MultiplyAdd10/3(in2)
  delayMatch57/1 -> _adder_MultiplyAdd11/1(in0)
  _adder_MultiplyAdd_out_dtc10/1 -> _adder_MultiplyAdd11/3(in2)
  _bias2/1 -> _adder_MultiplyAdd12/3(in2)
  delayMatch36/1 -> _adder_MultiplyAdd12/1(in0)
  t26/1 -> _adder_MultiplyAdd12/2(in1)
  delayMatch37/1 -> _adder_MultiplyAdd13/1(in0)
  _adder_MultiplyAdd_out_dtc12/1 -> _adder_MultiplyAdd13/3(in2)
  delayMatch38/1 -> _adder_MultiplyAdd14/1(in0)
  _adder_MultiplyAdd_out_dtc13/1 -> _adder_MultiplyAdd14/3(in2)
  delayMatch39/1 -> _adder_MultiplyAdd15/1(in0)
  _adder_MultiplyAdd_out_dtc14/1 -> _adder_MultiplyAdd15/3(in2)
  delayMatch40/1 -> _adder_MultiplyAdd16/1(in0)
  _adder_MultiplyAdd_out_dtc15/1 -> _adder_MultiplyAdd16/3(in2)
  delayMatch58/1 -> _adder_MultiplyAdd17/1(in0)
  _adder_MultiplyAdd_out_dtc16/1 -> _adder_MultiplyAdd17/3(in2)
  _bias3/1 -> _adder_MultiplyAdd18/3(in2)
  delayMatch41/1 -> _adder_MultiplyAdd18/1(in0)
  t28/1 -> _adder_MultiplyAdd18/2(in1)
  delayMatch42/1 -> _adder_MultiplyAdd19/1(in0)
  _adder_MultiplyAdd_out_dtc18/1 -> _adder_MultiplyAdd19/3(in2)
  delayMatch43/1 -> _adder_MultiplyAdd20/1(in0)
  _adder_MultiplyAdd_out_dtc19/1 -> _adder_MultiplyAdd20/3(in2)
  delayMatch44/1 -> _adder_MultiplyAdd21/1(in0)
  _adder_MultiplyAdd_out_dtc20/1 -> _adder_MultiplyAdd21/3(in2)
  delayMatch45/1 -> _adder_MultiplyAdd22/1(in0)
  _adder_MultiplyAdd_out_dtc21/1 -> _adder_MultiplyAdd22/3(in2)
  delayMatch59/1 -> _adder_MultiplyAdd23/1(in0)
  _adder_MultiplyAdd_out_dtc22/1 -> _adder_MultiplyAdd23/3(in2)
  _bias4/1 -> _adder_MultiplyAdd24/3(in2)
  delayMatch46/1 -> _adder_MultiplyAdd24/1(in0)
  t30/1 -> _adder_MultiplyAdd24/2(in1)
  delayMatch47/1 -> _adder_MultiplyAdd25/1(in0)
  _adder_MultiplyAdd_out_dtc24/1 -> _adder_MultiplyAdd25/3(in2)
  delayMatch48/1 -> _adder_MultiplyAdd26/1(in0)
  _adder_MultiplyAdd_out_dtc25/1 -> _adder_MultiplyAdd26/3(in2)
  delayMatch49/1 -> _adder_MultiplyAdd27/1(in0)
  _adder_MultiplyAdd_out_dtc26/1 -> _adder_MultiplyAdd27/3(in2)
  delayMatch50/1 -> _adder_MultiplyAdd28/1(in0)
  _adder_MultiplyAdd_out_dtc27/1 -> _adder_MultiplyAdd28/3(in2)
  delayMatch60/1 -> _adder_MultiplyAdd29/1(in0)
  _adder_MultiplyAdd_out_dtc28/1 -> _adder_MultiplyAdd29/3(in2)
  _bias5/1 -> _adder_MultiplyAdd30/3(in2)
  delayMatch51/1 -> _adder_MultiplyAdd30/1(in0)
  t32/1 -> _adder_MultiplyAdd30/2(in1)
  delayMatch52/1 -> _adder_MultiplyAdd31/1(in0)
  _adder_MultiplyAdd_out_dtc30/1 -> _adder_MultiplyAdd31/3(in2)
  delayMatch53/1 -> _adder_MultiplyAdd32/1(in0)
  _adder_MultiplyAdd_out_dtc31/1 -> _adder_MultiplyAdd32/3(in2)
  delayMatch54/1 -> _adder_MultiplyAdd33/1(in0)
  _adder_MultiplyAdd_out_dtc32/1 -> _adder_MultiplyAdd33/3(in2)
  delayMatch55/1 -> _adder_MultiplyAdd34/1(in0)
  _adder_MultiplyAdd_out_dtc33/1 -> _adder_MultiplyAdd34/3(in2)
  delayMatch61/1 -> _adder_MultiplyAdd35/1(in0)
  _adder_MultiplyAdd_out_dtc34/1 -> _adder_MultiplyAdd35/3(in2)
  Gain_const/1 -> Gain/1(in0)
  Gain2_const/1 -> Gain2/2(in1)
  Gain2_const1/1 -> Gain21/2(in1)
  Product_C2ReIm_1/1 -> Product/1(in0), Product1/1(in0)
  Product_C2ReIm_1/2 -> Product2/1(in0), Product3/1(in0)
  delayMatch16/1 -> Product/2(in1)
  delayMatch17/1 -> Product1/2(in1)
  Product/1(out0) -> Product_AC_minus_BD/1
  Product1/1(out0) -> Product_AD_plus_BC/1
  Product2/1(out0) -> Product_AC_minus_BD/2
  Product3/1(out0) -> Product_AD_plus_BC/2
  Product_AC_minus_BD/1 -> Product_ReIm2Complex/1
  Product_AD_plus_BC/1 -> Product_ReIm2Complex/2
  Product_C2ReIm_11/1 -> Product4/1(in0), Product5/1(in0)
  Product_C2ReIm_11/2 -> Product6/1(in0), Product7/1(in0)
  delayMatch21/1 -> Product4/2(in1)
  delayMatch22/1 -> Product5/2(in1)
  Product4/1(out0) -> Product_AC_minus_BD1/1
  Product5/1(out0) -> Product_AD_plus_BC1/1
  Product6/1(out0) -> Product_AC_minus_BD1/2
  Product7/1(out0) -> Product_AD_plus_BC1/2
  Product_AC_minus_BD1/1 -> Product_ReIm2Complex1/1
  Product_AD_plus_BC1/1 -> Product_ReIm2Complex1/2
  MMul_dot_product/1(out0) -> MMul_dot_product_out_dtc/1
  MMul_dot_product1/1(out0) -> MMul_dot_product_out_dtc1/1
  MMul_dot_product2/1(out0) -> MMul_dot_product_out_dtc2/1
  MMul_dot_product3/1(out0) -> MMul_dot_product_out_dtc3/1
  _adder_MultiplyAdd/1(out0) -> _adder_MultiplyAdd_out_dtc/1
  _adder_MultiplyAdd1/1(out0) -> _adder_MultiplyAdd_out_dtc1/1
  _adder_MultiplyAdd2/1(out0) -> _adder_MultiplyAdd_out_dtc2/1
  _adder_MultiplyAdd3/1(out0) -> _adder_MultiplyAdd_out_dtc3/1
  _adder_MultiplyAdd4/1(out0) -> _adder_MultiplyAdd_out_dtc4/1
  _adder_MultiplyAdd5/1(out0) -> _adder_MultiplyAdd_out_dtc5/1
  _adder_MultiplyAdd6/1(out0) -> _adder_MultiplyAdd_out_dtc6/1
  _adder_MultiplyAdd7/1(out0) -> _adder_MultiplyAdd_out_dtc7/1
  _adder_MultiplyAdd8/1(out0) -> _adder_MultiplyAdd_out_dtc8/1
  _adder_MultiplyAdd9/1(out0) -> _adder_MultiplyAdd_out_dtc9/1
  _adder_MultiplyAdd10/1(out0) -> _adder_MultiplyAdd_out_dtc10/1
  _adder_MultiplyAdd11/1(out0) -> _adder_MultiplyAdd_out_dtc11/1
  _adder_MultiplyAdd12/1(out0) -> _adder_MultiplyAdd_out_dtc12/1
  _adder_MultiplyAdd13/1(out0) -> _adder_MultiplyAdd_out_dtc13/1
  _adder_MultiplyAdd14/1(out0) -> _adder_MultiplyAdd_out_dtc14/1
  _adder_MultiplyAdd15/1(out0) -> _adder_MultiplyAdd_out_dtc15/1
  _adder_MultiplyAdd16/1(out0) -> _adder_MultiplyAdd_out_dtc16/1
  _adder_MultiplyAdd17/1(out0) -> _adder_MultiplyAdd_out_dtc17/1
  _adder_MultiplyAdd18/1(out0) -> _adder_MultiplyAdd_out_dtc18/1
  _adder_MultiplyAdd19/1(out0) -> _adder_MultiplyAdd_out_dtc19/1
  _adder_MultiplyAdd20/1(out0) -> _adder_MultiplyAdd_out_dtc20/1
  _adder_MultiplyAdd21/1(out0) -> _adder_MultiplyAdd_out_dtc21/1
  _adder_MultiplyAdd22/1(out0) -> _adder_MultiplyAdd_out_dtc22/1
  _adder_MultiplyAdd23/1(out0) -> _adder_MultiplyAdd_out_dtc23/1
  _adder_MultiplyAdd24/1(out0) -> _adder_MultiplyAdd_out_dtc24/1
  _adder_MultiplyAdd25/1(out0) -> _adder_MultiplyAdd_out_dtc25/1
  _adder_MultiplyAdd26/1(out0) -> _adder_MultiplyAdd_out_dtc26/1
  _adder_MultiplyAdd27/1(out0) -> _adder_MultiplyAdd_out_dtc27/1
  _adder_MultiplyAdd28/1(out0) -> _adder_MultiplyAdd_out_dtc28/1
  _adder_MultiplyAdd29/1(out0) -> _adder_MultiplyAdd_out_dtc29/1
  _adder_MultiplyAdd30/1(out0) -> _adder_MultiplyAdd_out_dtc30/1
  _adder_MultiplyAdd31/1(out0) -> _adder_MultiplyAdd_out_dtc31/1
  _adder_MultiplyAdd32/1(out0) -> _adder_MultiplyAdd_out_dtc32/1
  _adder_MultiplyAdd33/1(out0) -> _adder_MultiplyAdd_out_dtc33/1
  _adder_MultiplyAdd34/1(out0) -> _adder_MultiplyAdd_out_dtc34/1
  _adder_MultiplyAdd35/1(out0) -> _adder_MultiplyAdd_out_dtc35/1
  Gain2/1(out0) -> Gain2_out_dtc/1
  Gain21/1(out0) -> Gain2_out_dtc1/1
  delayMatch3/1 -> Divide2/2(in1)
  x_in_dq_0_wire/1 -> delayMatch3/1, delayMatch2/1
  delayMatch5/1 -> Divide3/2(in1)
  x_in_dq_1_wire/1 -> delayMatch5/1, delayMatch4/1
  t18/1(out0) -> delayMatch10/1
  t18/2(out1) -> delayMatch11/1
  t18/3(out2) -> delayMatch12/1
  t18/4(out3) -> delayMatch13/1
  t18/5(out4) -> delayMatch14/1
  t18/6(out5) -> delayMatch15/1
  delayMatch19/1 -> Product3/2(in1)
  delayMatch18/1 -> Product2/2(in1)
  Product_C2ReIm_2/2 -> delayMatch18/1, delayMatch17/1
  Product_C2ReIm_2/1 -> delayMatch19/1, delayMatch16/1
  Row2Col_in01/1 -> delayMatch20/1
  delayMatch24/1 -> Product7/2(in1)
  delayMatch23/1 -> Product6/2(in1)
  Product_C2ReIm_21/2 -> delayMatch23/1, delayMatch22/1
  Product_C2ReIm_21/1 -> delayMatch24/1, delayMatch21/1
  Row2Col_in03/1 -> delayMatch25/1
  t21/1 -> delayMatch26/1
  t21/2 -> delayMatch27/1
  t22/2 -> _adder_MultiplyAdd1/2(in1)
  t21/3 -> delayMatch28/1
  t22/3 -> _adder_MultiplyAdd2/2(in1)
  t21/4 -> delayMatch29/1
  t22/4 -> _adder_MultiplyAdd3/2(in1)
  t21/5 -> delayMatch30/1
  t22/5 -> _adder_MultiplyAdd4/2(in1)
  t23/1 -> delayMatch31/1
  t23/2 -> delayMatch32/1
  t24/2 -> _adder_MultiplyAdd7/2(in1)
  t23/3 -> delayMatch33/1
  t24/3 -> _adder_MultiplyAdd8/2(in1)
  t23/4 -> delayMatch34/1
  t24/4 -> _adder_MultiplyAdd9/2(in1)
  t23/5 -> delayMatch35/1
  t24/5 -> _adder_MultiplyAdd10/2(in1)
  t25/1 -> delayMatch36/1
  t25/2 -> delayMatch37/1
  t26/2 -> _adder_MultiplyAdd13/2(in1)
  t25/3 -> delayMatch38/1
  t26/3 -> _adder_MultiplyAdd14/2(in1)
  t25/4 -> delayMatch39/1
  t26/4 -> _adder_MultiplyAdd15/2(in1)
  t25/5 -> delayMatch40/1
  t26/5 -> _adder_MultiplyAdd16/2(in1)
  t27/1 -> delayMatch41/1
  t27/2 -> delayMatch42/1
  t28/2 -> _adder_MultiplyAdd19/2(in1)
  t27/3 -> delayMatch43/1
  t28/3 -> _adder_MultiplyAdd20/2(in1)
  t27/4 -> delayMatch44/1
  t28/4 -> _adder_MultiplyAdd21/2(in1)
  t27/5 -> delayMatch45/1
  t28/5 -> _adder_MultiplyAdd22/2(in1)
  t29/1 -> delayMatch46/1
  t29/2 -> delayMatch47/1
  t30/2 -> _adder_MultiplyAdd25/2(in1)
  t29/3 -> delayMatch48/1
  t30/3 -> _adder_MultiplyAdd26/2(in1)
  t29/4 -> delayMatch49/1
  t30/4 -> _adder_MultiplyAdd27/2(in1)
  t29/5 -> delayMatch50/1
  t30/5 -> _adder_MultiplyAdd28/2(in1)
  t31/1 -> delayMatch51/1
  t31/2 -> delayMatch52/1
  t32/2 -> _adder_MultiplyAdd31/2(in1)
  t31/3 -> delayMatch53/1
  t32/3 -> _adder_MultiplyAdd32/2(in1)
  t31/4 -> delayMatch54/1
  t32/4 -> _adder_MultiplyAdd33/2(in1)
  t31/5 -> delayMatch55/1
  t32/5 -> _adder_MultiplyAdd34/2(in1)
  t21/6 -> delayMatch56/1
  t22/6 -> _adder_MultiplyAdd5/2(in1)
  t23/6 -> delayMatch57/1
  t24/6 -> _adder_MultiplyAdd11/2(in1)
  t25/6 -> delayMatch58/1
  t26/6 -> _adder_MultiplyAdd17/2(in1)
  t27/6 -> delayMatch59/1
  t28/6 -> _adder_MultiplyAdd23/2(in1)
  t29/6 -> delayMatch60/1
  t30/6 -> _adder_MultiplyAdd29/2(in1)
  t31/6 -> delayMatch61/1
  t32/6 -> _adder_MultiplyAdd35/2(in1)
  From2/1 -> Divide/1(in0)
  From22/1 -> Divide31/1(in0)
  From3/1 -> Divide1/1(in0)
  From12/1 -> Divide21/1(in0)
  Demux1_mux_1/1 -> Demux1_out1/1
  Demux1_mux_2/1 -> Demux1_out2/1
  Switch/1 -> Switch_out1/1, Switch_out11/1
  enb_counter_ge_5_and_enb_counter_le_10/1 -> crp_temp_MAC1/Enable, crp_temp_MAC2/Enable, crp_temp_MAC/Enable, crp_temp_MAC3/Enable, crp_temp_MAC5/Enable, crp_temp_MAC4/Enable
  enb_counter_ge_26_and_enb_counter_le_28/1 -> Divide/Enable, Divide1/Enable, Divide31/Enable, Divide21/Enable
  enb_counter_ge_3_and_enb_counter_le_5/1 -> Divide4/Enable, Divide11/Enable, Divide2/Enable, Divide3/Enable
  enb_counter_le_2/1 -> Gain/Enable, MMul_dot_product2/Enable, MMul_dot_product/Enable
  enb_counter_ge_6_and_enb_counter_le_8/1 -> MMul_dot_product1/Enable, MMul_dot_product3/Enable
  enb_counter_ge_8_and_enb_counter_le_11/1 -> _adder_MultiplyAdd/Enable, _adder_MultiplyAdd6/Enable, _adder_MultiplyAdd12/Enable, _adder_MultiplyAdd18/Enable, _adder_MultiplyAdd24/Enable, _adder_MultiplyAdd30/Enable
  enb_counter_ge_11_and_enb_counter_le_14/1 -> _adder_MultiplyAdd1/Enable, _adder_MultiplyAdd7/Enable, _adder_MultiplyAdd13/Enable, _adder_MultiplyAdd19/Enable, _adder_MultiplyAdd25/Enable, _adder_MultiplyAdd31/Enable
  enb_counter_ge_14_and_enb_counter_le_17/1 -> _adder_MultiplyAdd2/Enable, _adder_MultiplyAdd8/Enable, _adder_MultiplyAdd14/Enable, _adder_MultiplyAdd20/Enable, _adder_MultiplyAdd26/Enable, _adder_MultiplyAdd32/Enable
  enb_counter_ge_17_and_enb_counter_le_20/1 -> _adder_MultiplyAdd3/Enable, _adder_MultiplyAdd9/Enable, _adder_MultiplyAdd15/Enable, _adder_MultiplyAdd21/Enable, _adder_MultiplyAdd27/Enable, _adder_MultiplyAdd33/Enable
  enb_counter_ge_20_and_enb_counter_le_23/1 -> _adder_MultiplyAdd4/Enable, _adder_MultiplyAdd10/Enable, _adder_MultiplyAdd16/Enable, _adder_MultiplyAdd22/Enable, _adder_MultiplyAdd28/Enable, _adder_MultiplyAdd34/Enable
  enb_counter_ge_23_and_enb_counter_le_26/1 -> _adder_MultiplyAdd5/Enable, _adder_MultiplyAdd11/Enable, _adder_MultiplyAdd17/Enable, _adder_MultiplyAdd23/Enable, _adder_MultiplyAdd29/Enable, _adder_MultiplyAdd35/Enable
  enb_counter_ge_2_and_enb_counter_le_4/1 -> Gain21/Enable, Gain2/Enable
  enb_counter_ge_4_and_enb_counter_le_6/1 -> Product/Enable, Product2/Enable, Product1/Enable, Product3/Enable, Product4/Enable, Product6/Enable, Product5/Enable, Product7/Enable
  enb_counter_ge_2/1 -> enb_counter_ge_2_and_enb_counter_le_4/1
  enb_counter_le_4/1 -> enb_counter_ge_2_and_enb_counter_le_4/2
  enb_counter_ge_3/1 -> enb_counter_ge_3_and_enb_counter_le_5/1
  enb_counter_le_5/1 -> enb_counter_ge_3_and_enb_counter_le_5/2
  enb_counter_ge_4/1 -> enb_counter_ge_4_and_enb_counter_le_6/1
  enb_counter_le_6/1 -> enb_counter_ge_4_and_enb_counter_le_6/2
  enb_counter_ge_5/1 -> enb_counter_ge_5_and_enb_counter_le_10/1
  enb_counter_le_10/1 -> enb_counter_ge_5_and_enb_counter_le_10/2
  enb_counter_ge_6/1 -> enb_counter_ge_6_and_enb_counter_le_8/1
  enb_counter_le_8/1 -> enb_counter_ge_6_and_enb_counter_le_8/2
  enb_counter_ge_8/1 -> enb_counter_ge_8_and_enb_counter_le_11/1
  enb_counter_le_11/1 -> enb_counter_ge_8_and_enb_counter_le_11/2
  enb_counter_ge_11/1 -> enb_counter_ge_11_and_enb_counter_le_14/1
  enb_counter_le_14/1 -> enb_counter_ge_11_and_enb_counter_le_14/2
  enb_counter_ge_14/1 -> enb_counter_ge_14_and_enb_counter_le_17/1
  enb_counter_le_17/1 -> enb_counter_ge_14_and_enb_counter_le_17/2
  enb_counter_ge_17/1 -> enb_counter_ge_17_and_enb_counter_le_20/1
  enb_counter_le_20/1 -> enb_counter_ge_17_and_enb_counter_le_20/2
  enb_counter_ge_20/1 -> enb_counter_ge_20_and_enb_counter_le_23/1
  enb_counter_le_23/1 -> enb_counter_ge_20_and_enb_counter_le_23/2
  enb_counter_ge_23/1 -> enb_counter_ge_23_and_enb_counter_le_26/1
  enb_counter_le_26/1 -> enb_counter_ge_23_and_enb_counter_le_26/2
  enb_counter_ge_26/1 -> enb_counter_ge_26_and_enb_counter_le_28/1
  enb_counter_le_28/1 -> enb_counter_ge_26_and_enb_counter_le_28/2
  ctr_99/1 -> enb_counter_le_28/1, enb_counter_ge_26/1, enb_counter_le_26/1, enb_counter_ge_23/1, enb_counter_le_23/1, enb_counter_ge_20/1, enb_counter_le_20/1, enb_counter_ge_17/1, enb_counter_le_17/1, enb_counter_ge_14/1, enb_counter_le_14/1, enb_counter_ge_11/1, enb_counter_le_11/1, enb_counter_ge_8/1, enb_counter_le_8/1, enb_counter_ge_6/1, enb_counter_le_10/1, enb_counter_ge_5/1, enb_counter_le_6/1, enb_counter_ge_4/1, enb_counter_le_5/1, enb_counter_ge_3/1, enb_counter_le_4/1, enb_counter_ge_2/1, enb_counter_le_2/1

== system gm_uz_sixphase_VSD_transformation/Line-Line to Phase voltage/abc   to   alpha_beta_0 ==
  "a, b, c" : Inport  PortDimensions=3
  Gain2 : Gain  Gain=2/3  ParamDataTypeStr=fixdt(1,18,16)  SaturateOnIntegerOverflow=on  OutDataTypeStr=Inherit: Same as input
  Gain4 : Gain  Gain="[ 1   -0.5   -0.5; 0   0.5*sqrt(3)   -0.5*sqrt(3); 0.5  0.5  0.5 ]"  Multiplication=Matrix(K*u) (u vector)  ParamDataTypeStr=fixdt(1,18,16)  OutDataTypeStr=fixdt(1,27,16)  SaturateOnIntegerOverflow=on
  "alpha, beta, 0 " : Outport
  wires:
  Gain4/1 -> Gain2/1
  "a, b, c"/1 -> Gain4/1
  Gain2/1 -> "alpha, beta, 0 "/1

== system gm_uz_sixphase_VSD_transformation/Line-Line to Phase voltage/alpha_beta_0   to   abc ==
  "alpha, beta, 0  " : Inport  PortDimensions=3
  Gain4 : Gain  Gain="[ 1 0 1; -0.5   0.5*sqrt(3)  1; -0.5 -0.5*sqrt(3) 1 ]"  Multiplication=Matrix(K*u) (u vector)  ParamDataTypeStr=fixdt(1,18,16)  SaturateOnIntegerOverflow=on  OutDataTypeStr=Inherit: Same as input
  "a, b, c" : Outport
  wires:
  "alpha, beta, 0  "/1 -> Gain4/1
  Gain4/1 -> "a, b, c"/1

== system gm_uz_sixphase_VSD_transformation/Line-Line to Phase voltage1/abc   to   alpha_beta_0 ==
  "a, b, c" : Inport  PortDimensions=3
  Gain2 : Gain  Gain=2/3  ParamDataTypeStr=fixdt(1,18,16)  SaturateOnIntegerOverflow=on  OutDataTypeStr=Inherit: Same as input
  Gain4 : Gain  Gain="[ 1   -0.5   -0.5; 0   0.5*sqrt(3)   -0.5*sqrt(3); 0.5  0.5  0.5 ]"  Multiplication=Matrix(K*u) (u vector)  ParamDataTypeStr=fixdt(1,18,16)  OutDataTypeStr=fixdt(1,27,16)  SaturateOnIntegerOverflow=on
  "alpha, beta, 0 " : Outport
  wires:
  Gain2/1 -> "alpha, beta, 0 "/1
  "a, b, c"/1 -> Gain4/1
  Gain4/1 -> Gain2/1

== system gm_uz_sixphase_VSD_transformation/Line-Line to Phase voltage1/alpha_beta_0   to   abc ==
  "alpha, beta, 0  " : Inport  PortDimensions=3
  Gain4 : Gain  Gain="[ 1 0 1; -0.5   0.5*sqrt(3)  1; -0.5 -0.5*sqrt(3) 1 ]"  Multiplication=Matrix(K*u) (u vector)  ParamDataTypeStr=fixdt(1,18,16)  SaturateOnIntegerOverflow=on  OutDataTypeStr=Inherit: Same as input
  "a, b, c" : Outport
  wires:
  Gain4/1 -> "a, b, c"/1
  "alpha, beta, 0  "/1 -> Gain4/1

== system gm_uz_sixphase_VSD_transformation/abc_to_dq/Divide ==
  in0 : Inport  OutDataTypeStr=fixdt(1, 18, 16)  SampleTime=1e-10
  in1 : Inport  Port=2  OutDataTypeStr=fixdt(1, 27, 16)  SampleTime=1e-10
  globalSchedule : EnablePort  OutDataTypeStr=boolean
  Divide : Product  Inputs=**  OutDataTypeStr=fixdt(1, 27, 16)  SampleTime=1e-10
  HwModeRegister : Delay  DelayLength=double(1)  InitialCondition=0
  HwModeRegister1 : Delay  DelayLength=double(1)  InitialCondition=0
  PipelineRegister : Delay  DelayLength=double(1)  InitialCondition=0
  out0 : Outport  OutDataTypeStr=fixdt(1, 27, 16)  SampleTime=1e-10  InitialOutput=0
  wires:
  PipelineRegister/1 -> out0/1
  in0/1 -> HwModeRegister/1
  in1/1 -> HwModeRegister1/1
  Divide/1 -> PipelineRegister/1
  HwModeRegister/1 -> Divide/1
  HwModeRegister1/1 -> Divide/2

== system gm_uz_sixphase_VSD_transformation/abc_to_dq/Divide1 ==
  in0 : Inport  OutDataTypeStr=fixdt(1, 18, 16)  SampleTime=1e-10
  in1 : Inport  Port=2  OutDataTypeStr=fixdt(1, 27, 16)  SampleTime=1e-10
  globalSchedule : EnablePort  OutDataTypeStr=boolean
  Divide1 : Product  Inputs=**  OutDataTypeStr=fixdt(1, 27, 16)  SampleTime=1e-10
  HwModeRegister : Delay  DelayLength=double(1)  InitialCondition=0
  HwModeRegister1 : Delay  DelayLength=double(1)  InitialCondition=0
  PipelineRegister : Delay  DelayLength=double(1)  InitialCondition=0
  out0 : Outport  OutDataTypeStr=fixdt(1, 27, 16)  SampleTime=1e-10  InitialOutput=0
  wires:
  PipelineRegister/1 -> out0/1
  in0/1 -> HwModeRegister/1
  in1/1 -> HwModeRegister1/1
  Divide1/1 -> PipelineRegister/1
  HwModeRegister/1 -> Divide1/1
  HwModeRegister1/1 -> Divide1/2

== system gm_uz_sixphase_VSD_transformation/abc_to_dq/Divide11 ==
  in0 : Inport  OutDataTypeStr=fixdt(1, 18, 16)  SampleTime=1e-10
  in1 : Inport  Port=2  OutDataTypeStr=fixdt(1, 27, 18)  SampleTime=1e-10
  globalSchedule : EnablePort  OutDataTypeStr=boolean
  Divide1 : Product  Inputs=**  OutDataTypeStr=fixdt(1, 27, 18)  SampleTime=1e-10
  HwModeRegister : Delay  DelayLength=double(1)  InitialCondition=0
  HwModeRegister1 : Delay  DelayLength=double(1)  InitialCondition=0
  PipelineRegister : Delay  DelayLength=double(1)  InitialCondition=0
  out0 : Outport  OutDataTypeStr=fixdt(1, 27, 18)  SampleTime=1e-10  InitialOutput=0
  wires:
  PipelineRegister/1 -> out0/1
  in0/1 -> HwModeRegister/1
  in1/1 -> HwModeRegister1/1
  Divide1/1 -> PipelineRegister/1
  HwModeRegister/1 -> Divide1/1
  HwModeRegister1/1 -> Divide1/2

== system gm_uz_sixphase_VSD_transformation/abc_to_dq/Divide2 ==
  in0 : Inport  OutDataTypeStr=fixdt(1, 18, 16)  SampleTime=1e-10
  in1 : Inport  Port=2  OutDataTypeStr=fixdt(1, 27, 18)  SampleTime=1e-10
  globalSchedule : EnablePort  OutDataTypeStr=boolean
  Divide2 : Product  Inputs=**  OutDataTypeStr=fixdt(1, 27, 18)  SampleTime=1e-10
  HwModeRegister : Delay  DelayLength=double(1)  InitialCondition=0
  HwModeRegister1 : Delay  DelayLength=double(1)  InitialCondition=0
  PipelineRegister : Delay  DelayLength=double(1)  InitialCondition=0
  out0 : Outport  OutDataTypeStr=fixdt(1, 27, 18)  SampleTime=1e-10  InitialOutput=0
  wires:
  PipelineRegister/1 -> out0/1
  in0/1 -> HwModeRegister/1
  in1/1 -> HwModeRegister1/1
  Divide2/1 -> PipelineRegister/1
  HwModeRegister/1 -> Divide2/1
  HwModeRegister1/1 -> Divide2/2
